simulink model "Narnia_model_quadRwdFn"  (R2023b)
settings: Solver=VariableStepAuto  StartTime=0.0  StopTime=inf  FixedStep=1  RelTol=1e-3  EnableMultiTasking=on
undefined symbols (not defined in the file or in its folder): A, B, DiscIntNeverNeededParam, E, HeatLimit
libraries: simulink x3, rllib x1
settings Model: Creator=The MathWorks, Inc.  LastModifiedBy=hdt
settings SolverCC: AlgebraicLoopSolver=TrustRegion  MinimalZcImpactIntegration=on
settings DataIOCC: LimitDataPoints=on  SaveFormat=Array
settings OptimizationCC: ReuseModelBlockBuffer=off  LifeSpan=inf
settings DebuggingCC: UnconnectedInputMsg=warning  UnconnectedOutputMsg=warning  UnconnectedLineMsg=warning  SFUnexpectedBacktrackingDiag=warning  SFNoUnconditionalDefaultTransitionDiag=warning  SFExecutionAtInitializationDiag=none  ArithmeticOperatorsInVariantConditions=warning
settings HardwareCC: ProdBitPerPointer=32  ProdBitPerSizeT=32  ProdBitPerPtrDiffT=32  ProdLargestAtomicFloat=None  ProdIntDivRoundTo=Undefined  ProdEndianess=Unspecified  ProdWordSize=32  ProdHWDeviceType=32-bit Generic
settings ModelReferenceCC: EnableRefExpFcnMdlSchedulingChecks=on  PropagateSignalLabelsOutOfModel=off
settings SFSimCC: SimUseLocalCustomCode=off  CustomCodeUndefinedFunction=UseInterfaceOnly
settings RTWCC: RTWUseLocalCustomCode=off
settings CodeAppCC: StateflowObjectComments=on
settings GRTTargetCC: TargetLangStandard=C89/C90 (ANSI)
settings ConfigComp: CovMetricSettings=dw  CovSaveCumulativeToWorkspaceVar=on  CovSaveSingleToWorkspaceVar=on  CovExternalEMLEnable=off  CovSFcnEnable=off

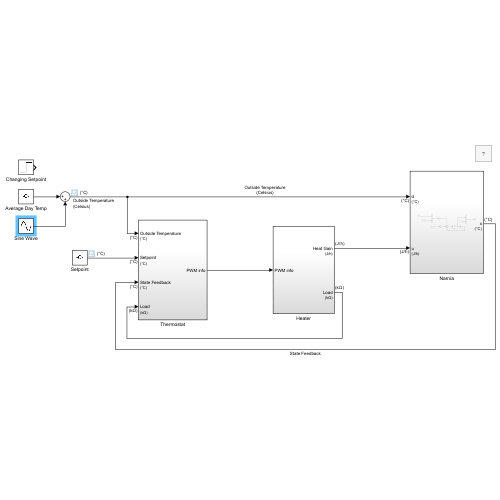
[thumbnail: Simulink's stored preview of the top-level diagram]
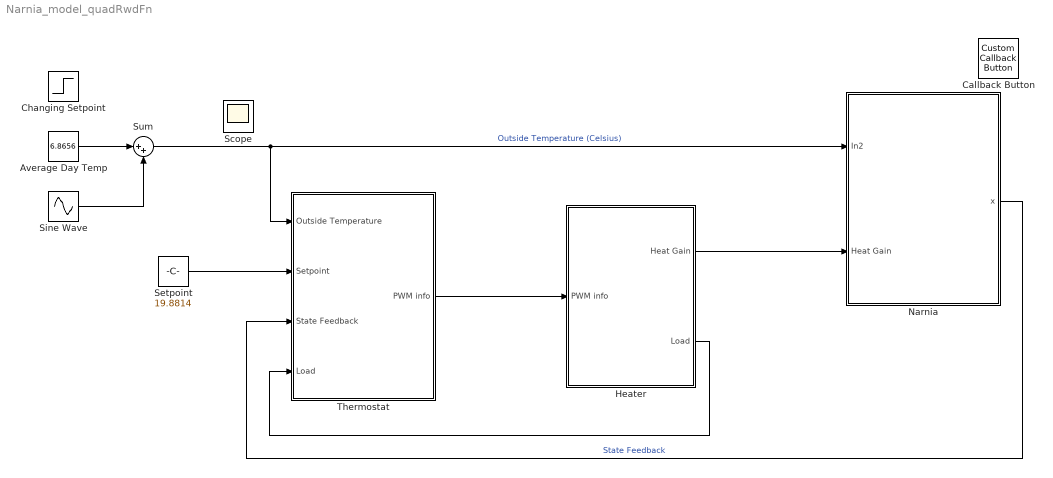
== system Narnia_model_quadRwdFn ==
  Average Day Temp : Constant  Value=6.8656
  Callback Button : CustomCallbackButton  Configuration="{\"components\":[{\"name\":\"BackgroundImageComponent\",\"settings\":{\"image\":{\"size\":[0,0],\"src\":\"default\",\"srcOrientation\":\"Right\"},\"position\":[0,0,1,1]}},{\"name\":\"ButtonStateComponent\",\"settings\":{\"buttonType\":\"momentary\",\"clickFcn\":\"showExample('simulink\\/OpenCompletedHouseSystemModelExample')\",\"onValue\":1,\"position\":[0,0,1,1],\"pressDelay\":\"500\",\"pressFcn\":\"\",\"repeatInterval\":\"0\",\"states\":[{\"horizontalAlignment\":\"center\",\"image\":{\"position\":[0,0,1,1],\"size\":[1,1],\"src\":\"default\",\"srcOrientation\":\"Right\"},\"label\":{\"color\":[0.01176470588,0.01176470588,0.01176470588,1],\"icon\":{\"size\":[0,0],\"src\":\"default\",\"srcOrientation\":\"Right\"},\"iconPlacement\":\"left\",\"opacity\":1,\"show\":true,\"text\":{\"content\":\"?\",\"font\":\"Helvetica\",\"fontSize\":14.735309999999998}},\"labelOffset\":[0,0],\"verticalAlignment\":\"middle\"},{\"horizontalAlignment\":\"center\",\"image\":{\"position\":[0,0,1,1],\"size\":[1,1],\"src\":\"default\",\"srcOrientation\":\"Right\"},\"label\":{\"color\":[0.01176470588,0.01176470588,0.01176470588,1],\"icon\":{\"size\":[0,0],\"src\":\"default\",\"srcOrientation\":\"Right\"},\"iconPlacement\":\"left\",\"opacity\":1,\"show\":true,\"text\":{\"content\":\"?\",\"font\":\"Helvetica\",\"fontSize\":14.735309999999998}},\"labelOffset\":[0,0],\"verticalAlignment\":\"middle\"},{\"horizontalAlignment\":\"center\",\"image\":{\"position\":[0,0,1,1],\"size\":[1,1],\"src\":\"default\",\"srcOrientation\":\"Right\"},\"label\":{\"color\":[0.01176470588,0.01176470588,0.01176470588,1],\"icon\":{\"size\":[0,0],\"src\":\"default\",\"srcOrientation\":\"Right\"},\"iconPlacement\":\"left\",\"opacity\":1,\"show\":true,\"text\":{\"content\":\"?\",\"font\":\"Helvetica\",\"fontSize\":14.735309999999998}},\"labelOffset\":[0,0],\"verticalAlignment\":\"middle\"},{\"horizontalAlignment\":\"center\",\"image\":{\"position\":[0,0,1,1],\"size\":[1,1],\"src\":\"default\",\"srcOrientation\":\"Right\"},\"label\":{\"color\":[0.01176470588,0.01176470588,0.01176470588,1],\"icon\":{\"size\":[0,0],\"src\":\"default\",\"srcOrientation\":\"Right\"},\"iconPlacement\":\"left\",\"opacity\":1,\"show\":true,\"text\":{\"content\":\"?\",\"font\":\"Helvetica\",\"fontSize\":14.735309999999998}},\"labelOffset\":[0,0],\"verticalAlignment\":\"middle\"}]}},{\"name\":\"ForegroundImageComponent\",\"settings\":{\"image\":{\"size\":[0,0],\"src\":\"default\",\"srcOrientation\":\"Right\"},\"isForeground\":1,\"position\":[0,0,1,1]}}],\"settings\":{\"BindingType\":\"standalone\",\"backgroundColor\":[244,244,244,1],\"backgroundOffset\":0,\"backgroundOpacity\":1,\"fixedAspectRatio\":\"off\",\"foregroundColor\":[0.01176470588,0.01176470588,0.01176470588,1],\"migratedFromLegacy\":true,\"useBackgroundColor\":true,\"variant\":\"callback\",\"version\":\"R2023a\"},\"type\":\"Button\"}"  CustomBackgroundColor="{\"color\":[0.9568627451,0.9568627451,0.9568627451],\"show\":true}"
  Changing Setpoint : Step  SampleTime=0
  Heater : Subsystem
  Narnia : Subsystem
  Setpoint : Constant  Value=19.8814
  Sine Wave : Sin  Amplitude=4  Frequency=pi/12  SampleTime=0
  Sum : Sum  Inputs=|++
  Thermostat : Subsystem
  Scope : Scope
  wires:
  Thermostat/1(PWM info) -> Heater/1(PWM info)
  Heater/1(Heat Gain) -> Narnia/2(Heat Gain)
  Narnia/1(x) -> Thermostat/3(State Feedback)  "State Feedback"
  Setpoint/1 -> Thermostat/2(Setpoint)
  Sine Wave/1 -> Sum/2
  Average Day Temp/1 -> Sum/1
  Sum/1 -> Thermostat/1(Outside Temperature), Narnia/1(In2)  "Outside Temperature (Celsius)"
  Heater/2(Load) -> Thermostat/4(Load)

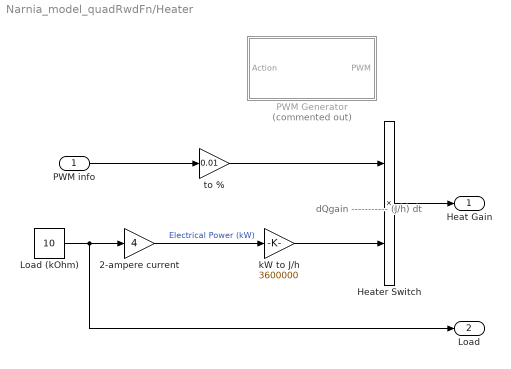
== system Narnia_model_quadRwdFn/Heater ==
  note: dQgain
      | ----------- (J/h)
      |    dt
  PWM info : Inport
  2-ampere current : Gain  Gain=4
  Heater Switch : Product  RndMeth=Zero
  Load (kOhm) : Constant  Value=10
  PWM Generator : Subsystem  Commented=on
  kW to J/h : Gain  Gain=3600000
  to % : Gain  Gain=0.01
  Heat Gain : Outport  Unit=joule/hour  VectorParamsAs1DForOutWhenUnconnected=off
  Load : Outport  Port=2  Unit=kΩ
  wires:
  Heater Switch/1 -> Heat Gain/1
  Load (kOhm)/1 -> Load/1, 2-ampere current/1
  kW to J/h/1 -> Heater Switch/2
  2-ampere current/1 -> kW to J/h/1  "Electrical Power (kW)"
  PWM info/1 -> to %/1
  to %/1 -> Heater Switch/1

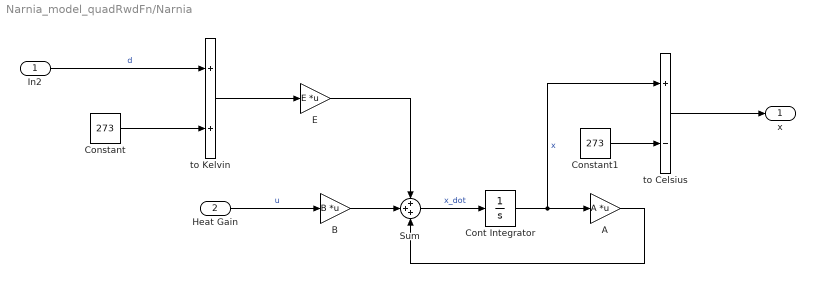
== system Narnia_model_quadRwdFn/Narnia ==
  In2 : Inport  Unit=Celsius
  Heat Gain : Inport  Port=2  Unit=J/h
  A : Gain  Gain=A  Multiplication=Matrix(K*u)
  B : Gain  Gain=B  Multiplication=Matrix(K*u)
  Constant : Constant  Value=273
  Constant1 : Constant  Value=273
  Cont Integrator : Integrator  InitialCondition=290.3332
  E : Gain  Gain=E  Multiplication=Matrix(K*u)
  Sum : Sum  Inputs=+++
  to Celsius : Sum  Inputs=+-
  to Kelvin : Sum
  x : Outport  Unit=°C
  wires:
  Heat Gain/1 -> B/1  "u"
  B/1 -> Sum/2
  A/1 -> Sum/3
  Sum/1 -> Cont Integrator/1  "x_dot"
  Cont Integrator/1 -> to Celsius/1, A/1  "x"
  E/1 -> Sum/1
  In2/1 -> to Kelvin/1  "d"
  Constant/1 -> to Kelvin/2
  to Kelvin/1 -> E/1
  to Celsius/1 -> x/1
  Constant1/1 -> to Celsius/2

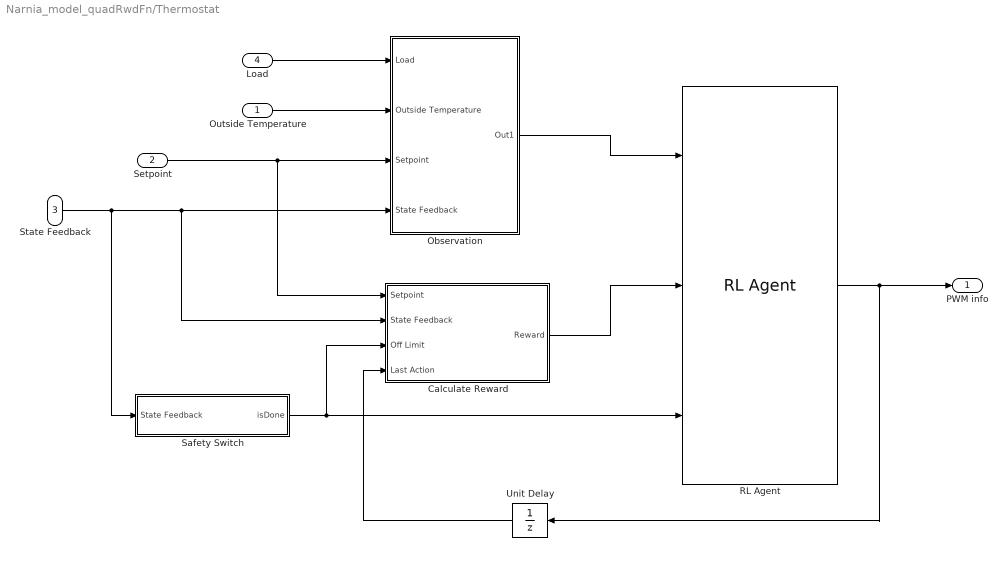
== system Narnia_model_quadRwdFn/Thermostat ==
  Outside Temperature : Inport  Unit=°C
  Setpoint : Inport  Port=2  Unit=°C
  State Feedback : Inport  Port=3  Unit=°C
  Load : Inport  Port=4  Unit=kΩ
  Calculate Reward : Subsystem
  Observation : Subsystem
  RL Agent : rllib/RL Agent  Agent=default_agent  ExternalActionAsInput=off  ProvideLastAction=off  ProvideCumRwd=off  TreatAsDirectFeedthrough=on  UseStrictObservationDataTypes=off
  Safety Switch : Subsystem
  Unit Delay : UnitDelay  SampleTime=-1  HasFrameUpgradeWarning=on
  PWM info : Outport  VectorParamsAs1DForOutWhenUnconnected=off
  wires:
  Setpoint/1 -> Calculate Reward/1(Setpoint), Observation/3(Setpoint)
  Outside Temperature/1 -> Observation/2(Outside Temperature)
  State Feedback/1 -> Calculate Reward/2(State Feedback), Observation/4(State Feedback), Safety Switch/1(State Feedback)
  Load/1 -> Observation/1(Load)
  RL Agent/1 -> Unit Delay/1, PWM info/1
  Observation/1(Out1) -> RL Agent/1
  Calculate Reward/1(Reward) -> RL Agent/2
  Safety Switch/1(isDone) -> RL Agent/3, Calculate Reward/3(Off Limit)
  Unit Delay/1 -> Calculate Reward/4(Last Action)

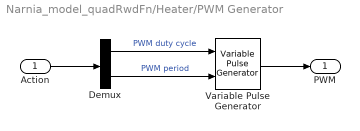
== system Narnia_model_quadRwdFn/Heater/PWM Generator ==
  Action : Inport
  Demux : Demux  Outputs=2
  Variable Pulse Generator : VariablePulseGenerator  AllowZeroPulseWidth=on  SampleTime=0.1
  PWM : Outport
  wires:
  Demux/1 -> Variable Pulse Generator/1  "PWM duty cycle"
  Demux/2 -> Variable Pulse Generator/2  "PWM period"
  Action/1 -> Demux/1
  Variable Pulse Generator/1 -> PWM/1

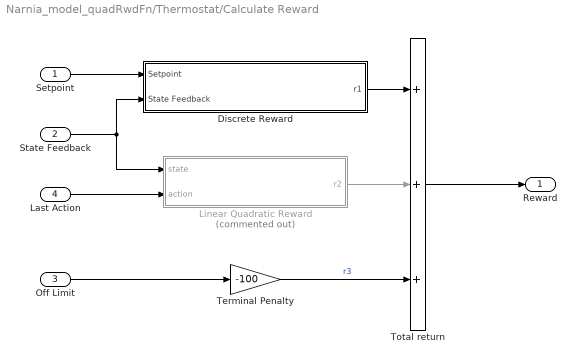
== system Narnia_model_quadRwdFn/Thermostat/Calculate Reward ==
  Setpoint : Inport
  State Feedback : Inport  Port=2
  Off Limit : Inport  Port=3
  Last Action : Inport  Port=4
  Discrete Reward : Subsystem
  Linear Quadratic Reward : Subsystem  Commented=on
  Terminal Penalty : Gain  Gain=-100
  Total return : Sum  Inputs=+++
  Reward : Outport
  wires:
  Total return/1 -> Reward/1
  Terminal Penalty/1 -> Total return/3  "r3"
  Off Limit/1 -> Terminal Penalty/1
  State Feedback/1 -> Discrete Reward/2(State Feedback), Linear Quadratic Reward/1(state)
  Linear Quadratic Reward/1(r2) -> Total return/2
  Last Action/1 -> Linear Quadratic Reward/2(action)
  Setpoint/1 -> Discrete Reward/1(Setpoint)
  Discrete Reward/1(r1) -> Total return/1

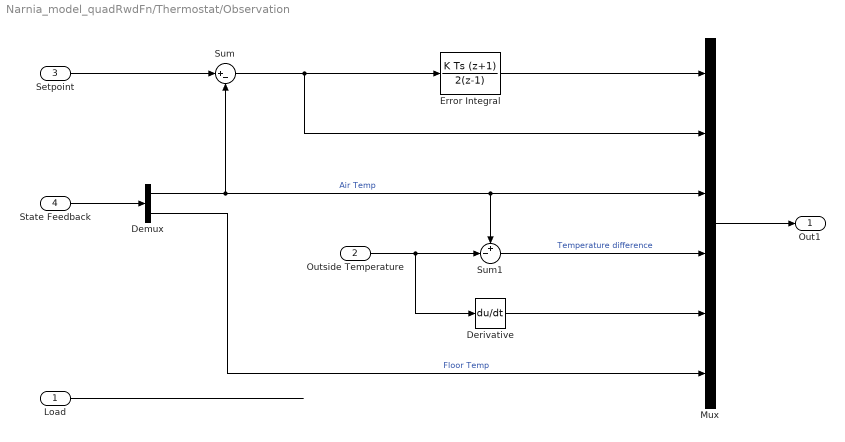
== system Narnia_model_quadRwdFn/Thermostat/Observation ==
  Load : Inport
  Outside Temperature : Inport  Port=2
  Setpoint : Inport  Port=3
  State Feedback : Inport  Port=4
  Demux : Demux  Outputs=2
  Derivative : Derivative
  Error Integral : DiscreteIntegrator  IntegratorMethod=Integration: Trapezoidal  SampleTime=-1  ICPrevOutput=DiscIntNeverNeededParam  ICPrevScaledInput=DiscIntNeverNeededParam
  Mux : Mux  Inputs=6
  Sum : Sum  Inputs=|+-
  Sum1 : Sum  Inputs=+-|
  Out1 : Outport
  wires:
  Outside Temperature/1 -> Derivative/1, Sum1/2
  Setpoint/1 -> Sum/1
  Demux/1 -> Sum/2, Sum1/1, Mux/3  "Air Temp"
  Error Integral/1 -> Mux/1
  Mux/1 -> Out1/1
  Sum/1 -> Mux/2, Error Integral/1
  Sum1/1 -> Mux/4  "Temperature difference"
  Load/1 -> ?
  State Feedback/1 -> Demux/1
  Demux/2 -> Mux/6  "Floor Temp"
  Derivative/1 -> Mux/5

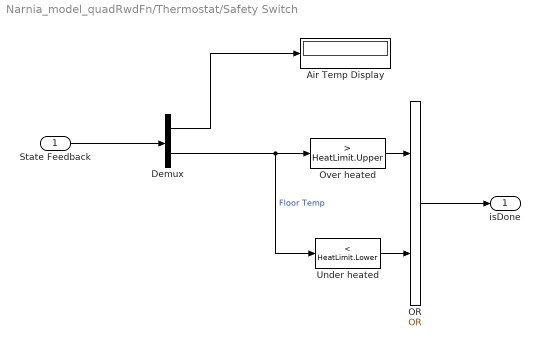
== system Narnia_model_quadRwdFn/Thermostat/Safety Switch ==
  State Feedback : Inport
  Air Temp Display : Display
  Demux : Demux  Outputs=2
  OR : Logic  Operator=OR  IconShape=distinctive  AllPortsSameDT=off  OutDataTypeStr=boolean
  Over heated : simulink/Logic and Bit Operations/Compare To Constant  relop=>  const=HeatLimit.Upper  OutDataTypeStr=boolean
  Under heated : simulink/Logic and Bit Operations/Compare To Constant  relop=<  const=HeatLimit.Lower  OutDataTypeStr=boolean
  isDone : Outport
  wires:
  Demux/2 -> Under heated/1, Over heated/1  "Floor Temp"
  Under heated/1 -> OR/2
  Over heated/1 -> OR/1
  OR/1 -> isDone/1
  Demux/1 -> Air Temp Display/1
  State Feedback/1 -> Demux/1

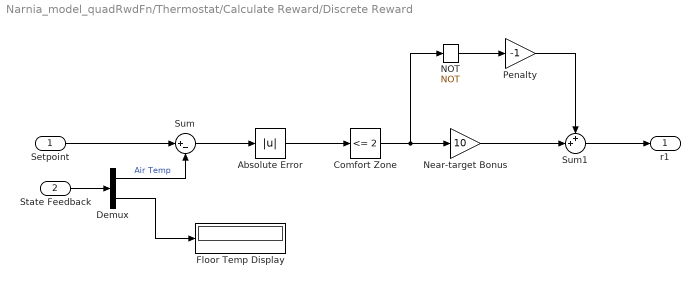
== system Narnia_model_quadRwdFn/Thermostat/Calculate Reward/Discrete Reward ==
  Setpoint : Inport
  State Feedback : Inport  Port=2
  Absolute Error : Abs  SaturateOnIntegerOverflow=off
  Comfort Zone : simulink/Logic and Bit Operations/Compare To Constant  relop=<=  const=2  OutDataTypeStr=boolean
  Demux : Demux  Outputs=2
  Floor Temp Display : Display
  NOT : Logic  Operator=NOT  IconShape=distinctive  AllPortsSameDT=off  OutDataTypeStr=boolean
  Near-target Bonus : Gain  Gain=10
  Penalty : Gain  Gain=-1
  Sum : Sum  Inputs=|+-
  Sum1 : Sum  Inputs=++|
  r1 : Outport
  wires:
  Setpoint/1 -> Sum/1
  State Feedback/1 -> Demux/1
  Near-target Bonus/1 -> Sum1/2
  Demux/2 -> Floor Temp Display/1
  Sum/1 -> Absolute Error/1
  Absolute Error/1 -> Comfort Zone/1
  Comfort Zone/1 -> NOT/1, Near-target Bonus/1
  Demux/1 -> Sum/2  "Air Temp"
  NOT/1 -> Penalty/1
  Penalty/1 -> Sum1/1
  Sum1/1 -> r1/1

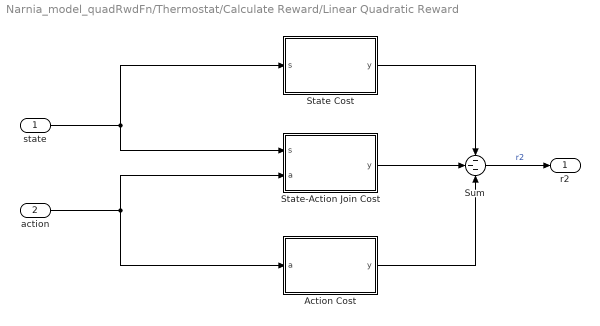
== system Narnia_model_quadRwdFn/Thermostat/Calculate Reward/Linear Quadratic Reward ==
  state : Inport
  action : Inport  Port=2
  Action Cost : MATLAB Function  TreatAsAtomicUnit=on
  State Cost : MATLAB Function  TreatAsAtomicUnit=on
  State-Action Join Cost : MATLAB Function  TreatAsAtomicUnit=on
  Sum : Sum  Inputs=---
  r2 : Outport
  wires:
  state/1 -> State Cost/1(s), State-Action Join Cost/1(s)
  action/1 -> State-Action Join Cost/2(a), Action Cost/1(a)
  State-Action Join Cost/1(y) -> Sum/2
  Action Cost/1(y) -> Sum/3
  Sum/1 -> r2/1  "r2"
  State Cost/1(y) -> Sum/1

== matlab function Narnia_model_quadRwdFn/Thermostat/Calculate Reward/Linear Quadratic Reward/State Cost ==
  data: s input; y output
function y = fcn(s)
    y = s'*QuadraticGains.Q*s;
end

== matlab function Narnia_model_quadRwdFn/Thermostat/Calculate Reward/Linear Quadratic Reward/State-Action Join Cost ==
  data: s input; a input; y output
function y = fcn(s, a)
    y = 2*s'*QuadraticGains.N*a;
end

== matlab function Narnia_model_quadRwdFn/Thermostat/Calculate Reward/Linear Quadratic Reward/Action Cost ==
  data: a input; y output
function y = fcn(a)
    y = a'*QuadraticGains.R*a;
end
